simulink model "CLAHEExample"  (R2019b)
settings: Solver=FixedStepDiscrete  StartTime=0.0  StopTime=402*324  FixedStep=1  RelTol=1e-3
PreLoadFcn:
  | % Initialize input image size
  | img = [240 320];
  | 
  | % Number of tiles fixed to 8 x 8
  | numTiles = [8 8];
  | 
  | % Initialize clip limit
  | normClipLimit  = 0.01;
  | 
  | % Number of Bins
  | numBins = 256;
  | 
  | dimI = [240 320] ;
  | 
  | dimTiles = dimI ./ numTiles;
  | 
  | numPixInTile = prod(dimTiles);
  | 
  | minClipLimit = ceil(numPixInTile/numBins);
  | 
  | clipLimit = minClipLimit + round(normClipLimit*(numPixInTile-minClipLimit));
  | 
  | % Initialize value for 1-D lookup table
  | tabVal = uint8(floor(numBins./(1:numBins-1)));
  | 
  | % Initialize wordlength and fractionlength
  | normFact1 = fi(1/(dimTiles(1)*dimTiles(2)/4),0);
  | 
  | normFact2 = fi(1/(prod(dimTiles)/2),0);
  | 
  | normFact3 = fi(1/(prod(dimTiles)),0);
  | 
  | grayxval = (numBins-1)/numPixInTile;
  | fi_grayxval = fi(grayxval,0);
InitFcn:
  | img = imread(get_param('CLAHEExample/inputImage','FileName'));
  | %img = [240 320];
  | numTiles = [8 8];
  | 
  | normClipLimit = str2double(get_param('CLAHEExample/CLAHEHDLAlgorithm','normClipLimit'));
  | 
  | numBins = 256;
  | 
  | dimI = size(img);
  | 
  | dimTiles = dimI ./ numTiles;
  | 
  | numPixInTile = prod(dimTiles);
  | 
  | minClipLimit = ceil(numPixInTile/numBins);
  | 
  | clipLimit = minClipLimit + round(normClipLimit*(numPixInTile-minClipLimit));
  | 
  | tabVal = uint8(floor(numBins./(1:numBins-1)));
  | 
  | normFact1 = fi(1/(dimTiles(1)*dimTiles(2)/4),0);
  | 
  | normFact2 = fi(1/(prod(dimTiles)/2),0);
  | 
  | normFact3 = fi(1/(prod(dimTiles)),0);
  | 
  | grayxval = (numBins-1)/numPixInTile;
  | fi_grayxval = fi(grayxval,0);
libraries: simulink x64, hdlsllib x46, visionhdlutilities x9, visionhdlstatistics x2, visionhdlio x2, visionsources x1
(part 1 of 3)
settings Model: SimulationMode=accelerator  Creator=The MathWorks, Inc.  LastModifiedBy=Bilal
settings OptimizationCC: BlockReduction=off  ConditionallyExecuteInputs=off  DefaultParameterBehavior=Inlined
settings DebuggingCC: AlgebraicLoopMsg=error  SymbolicDimsDataTypeCodeGenerationDiagnostic=none
settings HardwareCC: ProdBitPerPointer=32  ProdBitPerSizeT=32  ProdBitPerPtrDiffT=32  ProdLargestAtomicFloat=None  ProdIntDivRoundTo=Undefined  ProdEndianess=Unspecified  ProdWordSize=32  ProdHWDeviceType=ASIC/FPGA->ASIC/FPGA  TargetBitPerPointer=64  TargetBitPerSizeT=64  TargetBitPerPtrDiffT=64  TargetLongLongMode=on  TargetIntDivRoundTo=Zero  TargetEndianess=LittleEndian  TargetWordSize=64  TargetHWDeviceType=Custom Processor->MATLAB Host Computer  ProdEqTarget=off

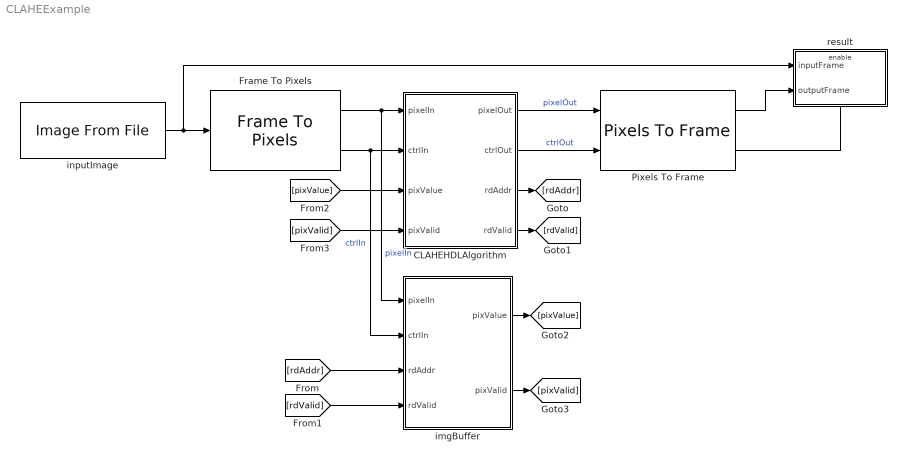
== system CLAHEExample ==
  CLAHEHDLAlgorithm : Subsystem  TreatAsAtomicUnit=on  mask{normClipLimit=0.01}
      mask prompts: normClipLimit "Normalized Clip Limit"
  Frame To Pixels : visionhdlio/Frame To Pixels  NumComponents=1  NumPixels=1  VideoFormat=240p  ActivePixelsPerLine=400  ActiveVideoLines=400  TotalPixelsPerLine=482  TotalVideoLines=430  StartingActiveLine=1  FrontPorch=41  SampleTime=0
      settings: SourceProductName=Vision HDL Toolbox  SourceProductBaseCode=VT
  Pixels To Frame : visionhdlio/Pixels To Frame  NumComponents=1  NumPixels=1  VideoFormat=240p  ActivePixelsPerLine=400  ActiveVideoLines=400  TotalPixelsPerLine=482  TotalVideoLines=430
      settings: SourceProductName=Vision HDL Toolbox  SourceProductBaseCode=VT
  imgBuffer : Subsystem
  inputImage : visionsources/Image From File  Tag=vipblks_nd  FileName=spine240p.tif  Ts=402*324  imagePorts=One multidimensional signal  OutPortLabels=R|G|B  ImageDataType=Inherit from input image  sdImageDataType=uint(8)  Signed=on  WordLength=16  FractionLengthMode=User-defined  FractionLength=15
      settings: SourceProductName=Computer Vision Toolbox
  result : Subsystem
  wires:
  CLAHEHDLAlgorithm/3(rdAddr) -> [rdAddr]
  [pixValue] -> CLAHEHDLAlgorithm/3(pixValue)
  CLAHEHDLAlgorithm/4(rdValid) -> [rdValid]
  inputImage/1 -> result/1(inputFrame), Frame To Pixels/1
  imgBuffer/1(pixValue) -> [pixValue]
  Frame To Pixels/2 -> CLAHEHDLAlgorithm/2(ctrlIn), imgBuffer/2(ctrlIn)  "ctrlIn"
  imgBuffer/2(pixValid) -> [pixValid]
  Pixels To Frame/1 -> result/2(outputFrame)
  CLAHEHDLAlgorithm/2(ctrlOut) -> Pixels To Frame/2  "ctrlOut"
  [pixValid] -> CLAHEHDLAlgorithm/4(pixValid)
  [rdAddr] -> imgBuffer/3(rdAddr)
  Frame To Pixels/1 -> CLAHEHDLAlgorithm/1(pixelIn), imgBuffer/1(pixelIn)  "pixelIn"
  Pixels To Frame/2 -> result/Enable
  [rdValid] -> imgBuffer/4("rdValid ")
  CLAHEHDLAlgorithm/1(pixelOut) -> Pixels To Frame/1  "pixelOut"

== system CLAHEExample/CLAHEHDLAlgorithm ==
  pixelIn : Inport
  ctrlIn : Inport  Port=2
  pixValue : Inport  Port=3
  pixValid : Inport  Port=4
  bilinearInterpolation : Subsystem
  busCreator : Subsystem
  histoEqPipeline : Subsystem
  tileGeneration : Subsystem
  pixelOut : Outport  VectorParamsAs1DForOutWhenUnconnected=off
  ctrlOut : Outport  Port=2  VectorParamsAs1DForOutWhenUnconnected=off
  rdAddr : Outport  Port=3  VectorParamsAs1DForOutWhenUnconnected=off
  rdValid : Outport  Port=4  VectorParamsAs1DForOutWhenUnconnected=off
  wires:
  tileGeneration/2(pixelOut) -> histoEqPipeline/2(pixelIn)
  tileGeneration/3(busPipeline1) -> histoEqPipeline/3(busPipeline1)
  tileGeneration/4(busPipeline2) -> histoEqPipeline/4(busPipeline2)
  tileGeneration/5(resetOut) -> histoEqPipeline/5(reset)
  ctrlIn/1 -> bilinearInterpolation/7(inputCtrl), tileGeneration/2(busIn)
  pixelIn/1 -> tileGeneration/1(pixelIn)
  histoEqPipeline/6(statePipe2) -> bilinearInterpolation/6(statePipe2)
  histoEqPipeline/5(cdfValidPipe2) -> bilinearInterpolation/5(cdfValidPipe2)
  histoEqPipeline/4(cdfValPipe2) -> bilinearInterpolation/4(cdfValPipe2)
  histoEqPipeline/3(statePipe1) -> bilinearInterpolation/3(statePipe1)
  histoEqPipeline/2(cdfValidPipe1) -> bilinearInterpolation/2(cdfValidPipe1)
  histoEqPipeline/1(cdfValPipe1) -> bilinearInterpolation/1(cdfValPipe1)
  bilinearInterpolation/4(pipe2Done) -> [pipe2]
  [pipe2] -> histoEqPipeline/7(state5Pipe2)
  bilinearInterpolation/3(pipe1Done) -> [pipe1]
  [pipe1] -> histoEqPipeline/6(state5Pipe1)
  bilinearInterpolation/5(rdAddr) -> rdAddr/1
  bilinearInterpolation/6(rdValid) -> rdValid/1
  pixValue/1 -> busCreator/1(rd_addr)
  pixValid/1 -> busCreator/2(rd_valid)
  busCreator/1(rdTile1) -> histoEqPipeline/8(state5Bus)
  tileGeneration/1(tileNumber) -> histoEqPipeline/1(tileNumber)
  bilinearInterpolation/1(CLAHEOut) -> pixelOut/1
  bilinearInterpolation/2(ctrlOut) -> ctrlOut/1
  bilinearInterpolation/7(frameDone) -> histoEqPipeline/9(frameDone)

== system CLAHEExample/imgBuffer ==
  pixelIn : Inport
  ctrlIn : Inport  Port=2
  rdAddr : Inport  Port=3
  "rdValid " : Inport  Port=4
  Bus Selector : BusSelector  OutputSignals=vStart,valid
  Delay : Delay  DelayLength=1
  Delay1 : Delay  DelayLength=1
  Delay2 : Delay  DelayLength=1
  HDL Counter : hdlsllib/Sources/HDL Counter  CountType=Count limited  CountInit=0  CountStep=1  CountMax=prod(dimI) - 1  CountFromType=Initial value  CountFrom=0  CountResetPort=on  CountLoadPort=off  CountEnbPort=on  CountDirPort=off  CountDataType=Unsigned  CountWordLen=ceil(log2(prod(dimI)))  CountFracLen=0  CountSampTime=1
      settings: SourceProductName=Simulink
  inputBuffer : hdlsllib/HDL RAMs/Simple Dual Port RAM System  RAMType=Simple dual port  WriteOutputValue=New data  RAMInitialValue=0  SimulateUsing=Code generation
      settings: SourceProductName=Simulink  SourceProductBaseCode=SL
  pixValue : Outport  VectorParamsAs1DForOutWhenUnconnected=off
  pixValid : Outport  Port=2  VectorParamsAs1DForOutWhenUnconnected=off
  wires:
  Delay1/1 -> inputBuffer/1
  Delay/1 -> inputBuffer/3, HDL Counter/2
  Bus Selector/1 -> HDL Counter/1  "<vStart>"
  HDL Counter/1 -> inputBuffer/2
  ctrlIn/1 -> Bus Selector/1
  Bus Selector/2 -> Delay/1  "<valid>"
  pixelIn/1 -> Delay1/1
  "rdValid "/1 -> Delay2/1
  rdAddr/1 -> inputBuffer/4
  inputBuffer/1 -> pixValue/1  "rd_addr"
  Delay2/1 -> pixValid/1  "rd_valid"

== system CLAHEExample/result ==
  inputFrame : Inport
  outputFrame : Inport  Port=2
  Enable : EnablePort
  Input Image : VideoViewer  FigPos=[579 574 378 287]
  Output Image : VideoViewer  FigPos=[579 573 378 285]
  wires:
  outputFrame/1 -> Output Image/1
  inputFrame/1 -> Input Image/1

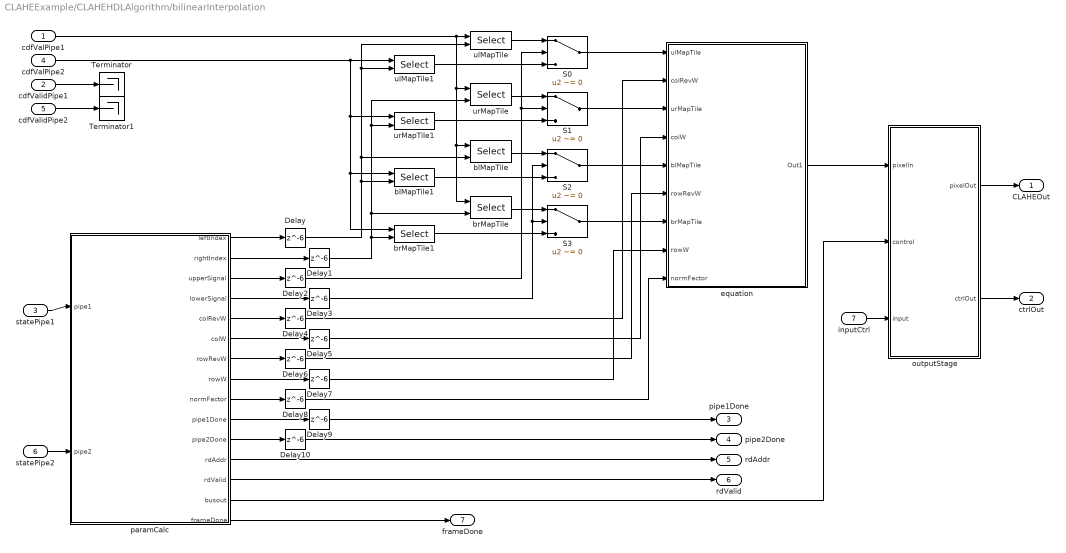
== system CLAHEExample/CLAHEHDLAlgorithm/bilinearInterpolation ==
  cdfValPipe1 : Inport
  cdfValidPipe1 : Inport  Port=2
  statePipe1 : Inport  Port=3
  cdfValPipe2 : Inport  Port=4
  cdfValidPipe2 : Inport  Port=5
  statePipe2 : Inport  Port=6
  inputCtrl : Inport  Port=7
  Delay : Delay  DelayLength=6  InitialCondition=1
  Delay1 : Delay  DelayLength=6  InitialCondition=1
  Delay{2..10} (9 alike) : Delay  DelayLength=6
  S{0..3} (4 alike) : Switch  Criteria=u2 ~= 0
  Terminator : Terminator
  Terminator1 : Terminator
  blMapTile : Selector  InputPortWidth=numTiles(2)  IndexOptions=Index vector (port)  Indices=[1 numTiles(2)]  OutputSizes=1
  blMapTile1 : Selector  InputPortWidth=numTiles(2)  IndexOptions=Index vector (port)  Indices=[1 numTiles(2)]  OutputSizes=1
  brMapTile : Selector  InputPortWidth=numTiles(2)  IndexOptions=Index vector (port)  Indices=[1 numTiles(2)]  OutputSizes=1
  brMapTile1 : Selector  InputPortWidth=numTiles(2)  IndexOptions=Index vector (port)  Indices=[1 numTiles(2)]  OutputSizes=1
  equation : Subsystem
  outputStage : Subsystem
  paramCalc : Subsystem
  ulMapTile : Selector  InputPortWidth=numTiles(2)  IndexOptions=Index vector (port)  Indices=[1 numTiles(2)]  OutputSizes=1
  ulMapTile1 : Selector  InputPortWidth=numTiles(2)  IndexOptions=Index vector (port)  Indices=[1 numTiles(2)]  OutputSizes=1
  urMapTile : Selector  InputPortWidth=numTiles(2)  IndexOptions=Index vector (port)  Indices=[1 numTiles(2)]  OutputSizes=1
  urMapTile1 : Selector  InputPortWidth=numTiles(2)  IndexOptions=Index vector (port)  Indices=[1 numTiles(2)]  OutputSizes=1
  CLAHEOut : Outport  VectorParamsAs1DForOutWhenUnconnected=off
  ctrlOut : Outport  Port=2  VectorParamsAs1DForOutWhenUnconnected=off
  pipe1Done : Outport  Port=3  VectorParamsAs1DForOutWhenUnconnected=off
  pipe2Done : Outport  Port=4  VectorParamsAs1DForOutWhenUnconnected=off
  rdAddr : Outport  Port=5  VectorParamsAs1DForOutWhenUnconnected=off
  rdValid : Outport  Port=6  VectorParamsAs1DForOutWhenUnconnected=off
  frameDone : Outport  Port=7  VectorParamsAs1DForOutWhenUnconnected=off
  wires:
  S0/1 -> equation/1(ulMapTile)
  S1/1 -> equation/3(urMapTile)
  S2/1 -> equation/5(blMapTile)
  S3/1 -> equation/7(brMapTile)
  urMapTile/1 -> S1/1
  ulMapTile/1 -> S0/1
  blMapTile/1 -> S2/1
  brMapTile/1 -> S3/1
  ulMapTile1/1 -> S0/3
  urMapTile1/1 -> S1/3
  blMapTile1/1 -> S2/3
  brMapTile1/1 -> S3/3
  cdfValPipe1/1 -> brMapTile/1, blMapTile/1, urMapTile/1, ulMapTile/1
  paramCalc/1(leftIndex) -> Delay/1
  paramCalc/2(rightIndex) -> Delay1/1
  paramCalc/3(upperSignal) -> Delay2/1
  paramCalc/4(lowerSignal) -> Delay3/1
  paramCalc/6(colW) -> Delay5/1
  paramCalc/5(colRevW) -> Delay4/1
  paramCalc/8(rowW) -> Delay7/1
  paramCalc/7(rowRevW) -> Delay6/1
  paramCalc/9(normFactor) -> Delay8/1
  statePipe1/1 -> paramCalc/1(pipe1)
  statePipe2/1 -> paramCalc/2(pipe2)
  paramCalc/10(pipe1Done) -> Delay9/1
  paramCalc/11(pipe2Done) -> Delay10/1
  paramCalc/12(rdAddr) -> rdAddr/1
  paramCalc/13(rdValid) -> rdValid/1
  cdfValidPipe2/1 -> Terminator1/1
  Delay/1 -> blMapTile1/2, blMapTile/2, ulMapTile1/2, ulMapTile/2
  Delay1/1 -> brMapTile/2, urMapTile/2, urMapTile1/2, brMapTile1/2
  Delay3/1 -> S3/2, S2/2
  Delay2/1 -> S1/2, S0/2
  Delay4/1 -> equation/2(colRevW)
  Delay5/1 -> equation/4(colW)
  Delay7/1 -> equation/8(rowW)
  Delay6/1 -> equation/6(rowRevW)
  Delay8/1 -> equation/9(normFactor)
  Delay10/1 -> pipe2Done/1
  Delay9/1 -> pipe1Done/1
  cdfValidPipe1/1 -> Terminator/1
  cdfValPipe2/1 -> brMapTile1/1, blMapTile1/1, urMapTile1/1, ulMapTile1/1
  inputCtrl/1 -> outputStage/3("input ")
  paramCalc/14(busout) -> outputStage/2("control ")
  paramCalc/15(frameDone) -> frameDone/1
  equation/1(Out1) -> outputStage/1(pixelIn)
  outputStage/1(pixelOut) -> CLAHEOut/1
  outputStage/2(ctrlOut) -> ctrlOut/1

== system CLAHEExample/CLAHEHDLAlgorithm/busCreator ==
  rd_addr : Inport
  rd_valid : Inport  Port=2
  Bus Creator : BusCreator  Inputs=5
  Constant : Constant  OutDataTypeStr=fixdt(0,ceil(log2(numPixInTile)),0)  SampleTime=-1
  Constant1 : Constant  Value=0  OutDataTypeStr=uint8  SampleTime=-1
  Constant2 : Constant  Value=0  OutDataTypeStr=boolean  SampleTime=-1
  rdTile1 : Outport  VectorParamsAs1DForOutWhenUnconnected=off
  wires:
  rd_addr/1 -> Bus Creator/4  "rd_addr"
  Constant1/1 -> Bus Creator/2  "wr_addr"
  Bus Creator/1 -> rdTile1/1
  Constant2/1 -> Bus Creator/3  "wr_en"
  Constant/1 -> Bus Creator/1  "histVal"
  rd_valid/1 -> Bus Creator/5  "rd_valid"

== system CLAHEExample/CLAHEHDLAlgorithm/histoEqPipeline ==
  tileNumber : Inport
  pixelIn : Inport  Port=2
  busPipeline1 : Inport  Port=3
  busPipeline2 : Inport  Port=4
  reset : Inport  Port=5
  state5Pipe1 : Inport  Port=6
  state5Pipe2 : Inport  Port=7
  state5Bus : Inport  Port=8
  frameDone : Inport  Port=9
  Constant : Constant  Value=1:numTiles(2)  OutDataTypeStr=uint8  SampleTime=-1
  histPipe1 : Subsystem  TreatAsAtomicUnit=on
  histPipe2 : Subsystem  TreatAsAtomicUnit=on
  cdfValPipe1 : Outport  VectorParamsAs1DForOutWhenUnconnected=off
  cdfValidPipe1 : Outport  Port=2  VectorParamsAs1DForOutWhenUnconnected=off
  statePipe1 : Outport  Port=3  VectorParamsAs1DForOutWhenUnconnected=off
  cdfValPipe2 : Outport  Port=4  VectorParamsAs1DForOutWhenUnconnected=off
  cdfValidPipe2 : Outport  Port=5  VectorParamsAs1DForOutWhenUnconnected=off
  statePipe2 : Outport  Port=6  VectorParamsAs1DForOutWhenUnconnected=off
  wires:
  pixelIn/1 -> histPipe2/3(pixelIn), histPipe1/3(pixelIn)
  reset/1 -> histPipe2/5(reset), histPipe1/5(reset)
  busPipeline1/1 -> histPipe1/4(busIn1)
  busPipeline2/1 -> histPipe2/4(busIn1)
  histPipe1/1(cdfVal) -> cdfValPipe1/1
  histPipe1/2(cdfValid) -> cdfValidPipe1/1
  histPipe1/3(pipeState) -> statePipe1/1
  histPipe2/3(pipeState) -> statePipe2/1
  state5Bus/1 -> histPipe1/7(state5Bus), histPipe2/7(state5Bus)
  state5Pipe1/1 -> histPipe1/6(state5Done)
  state5Pipe2/1 -> histPipe2/6(state5Done)
  tileNumber/1 -> histPipe2/2(tileNumber), histPipe1/2(tileNumber)
  Constant/1 -> histPipe2/1(index), histPipe1/1(index)
  frameDone/1 -> histPipe2/8(frameDone), histPipe1/8(frameDone)
  histPipe2/2(cdfValid) -> cdfValidPipe2/1
  histPipe2/1(cdfVal) -> cdfValPipe2/1

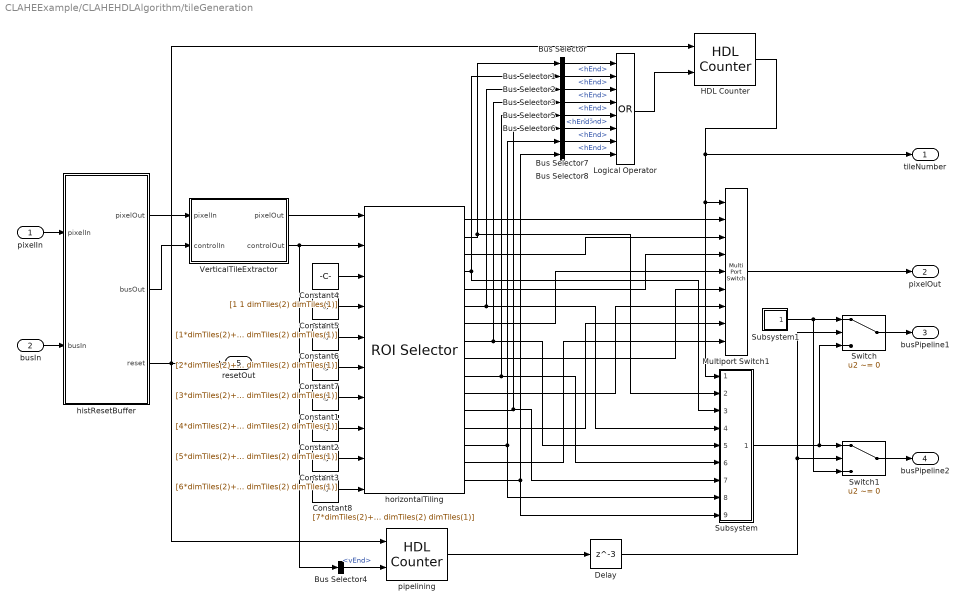
== system CLAHEExample/CLAHEHDLAlgorithm/tileGeneration ==
  pixelIn : Inport
  busIn : Inport  Port=2
  Bus Selector{,1..3,5..8} (8 alike) : BusSelector  OutputSignals=hEnd
  Bus Selector4 : BusSelector  OutputSignals=vEnd
  Constant1 : Constant  Value=[4*dimTiles(2)+1 1 dimTiles(2) dimTiles(1)]  OutDataTypeStr=fixdt(0,ceil(log2(dimI(2))),0)  SampleTime=-1
  Constant2 : Constant  Value=[5*dimTiles(2)+1 1 dimTiles(2) dimTiles(1)]  OutDataTypeStr=fixdt(0,ceil(log2(dimI(2))),0)  SampleTime=-1
  Constant3 : Constant  Value=[6*dimTiles(2)+1 1 dimTiles(2) dimTiles(1)]  OutDataTypeStr=fixdt(0,ceil(log2(dimI(2))),0)  SampleTime=-1
  Constant4 : Constant  Value=[1 1 dimTiles(2) dimTiles(1)]  OutDataTypeStr=fixdt(0,ceil(log2(dimI(2))),0)  SampleTime=-1
  Constant5 : Constant  Value=[1*dimTiles(2)+1 1 dimTiles(2) dimTiles(1)]  OutDataTypeStr=fixdt(0,ceil(log2(dimI(2))),0)  SampleTime=-1
  Constant6 : Constant  Value=[2*dimTiles(2)+1 1 dimTiles(2) dimTiles(1)]  OutDataTypeStr=fixdt(0,ceil(log2(dimI(2))),0)  SampleTime=-1
  Constant7 : Constant  Value=[3*dimTiles(2)+1 1 dimTiles(2) dimTiles(1)]  OutDataTypeStr=fixdt(0,ceil(log2(dimI(2))),0)  SampleTime=-1
  Constant8 : Constant  Value=[7*dimTiles(2)+1 1 dimTiles(2) dimTiles(1)]  OutDataTypeStr=fixdt(0,ceil(log2(dimI(2))),0)  SampleTime=-1
  Delay : Delay  DelayLength=3
  HDL Counter : hdlsllib/Sources/HDL Counter  CountType=Count limited  CountInit=1  CountStep=1  CountMax=numTiles(2)  CountFromType=Initial value  CountFrom=1  CountResetPort=on  CountLoadPort=off  CountEnbPort=on  CountDirPort=off  CountDataType=Unsigned  CountWordLen=4  CountFracLen=0  CountSampTime=1
      settings: SourceProductName=Simulink
  Logical Operator : Logic  Operator=OR  Inputs=8  AllPortsSameDT=off  OutDataTypeStr=boolean
  Multiport Switch1 : MultiPortSwitch  Inputs=8
  Subsystem : Subsystem
  Subsystem1 : Subsystem
  Switch : Switch  Criteria=u2 ~= 0
  Switch1 : Switch  Criteria=u2 ~= 0
  VerticalTileExtractor : Subsystem
  histResetBuffer : Subsystem
  horizontalTiling : visionhdlutilities/ROI Selector  RegionsSource=Input port  NumberOfRegions=8  Regions=[100 100 50 50]  SimulateUsing=Code generation
      settings: SourceProductName=Vision HDL Toolbox  SourceProductBaseCode=VT
  pipelining : hdlsllib/Sources/HDL Counter  CountType=Count limited  CountInit=0  CountStep=1  CountMax=1  CountFromType=Initial value  CountFrom=0  CountResetPort=on  CountLoadPort=off  CountEnbPort=on  CountDirPort=off  CountDataType=Unsigned  CountWordLen=4  CountFracLen=0  CountSampTime=1
      settings: SourceProductName=Simulink
  tileNumber : Outport  VectorParamsAs1DForOutWhenUnconnected=off
  pixelOut : Outport  Port=2  VectorParamsAs1DForOutWhenUnconnected=off
  busPipeline1 : Outport  Port=3  VectorParamsAs1DForOutWhenUnconnected=off
  busPipeline2 : Outport  Port=4  VectorParamsAs1DForOutWhenUnconnected=off
  resetOut : Outport  Port=5  VectorParamsAs1DForOutWhenUnconnected=off
  wires:
  pixelIn/1 -> histResetBuffer/1(pixelIn)
  busIn/1 -> histResetBuffer/2(busIn)
  VerticalTileExtractor/2(controlOut) -> Bus Selector4/1, horizontalTiling/2
  Constant6/1 -> horizontalTiling/5
  Constant4/1 -> horizontalTiling/3
  Constant7/1 -> horizontalTiling/6
  Constant5/1 -> horizontalTiling/4
  histResetBuffer/1(pixelOut) -> VerticalTileExtractor/1(pixelIn)
  histResetBuffer/2(busOut) -> VerticalTileExtractor/2(controlIn)
  HDL Counter/1 -> tileNumber/1, Subsystem/1(In1), Multiport Switch1/1
  Logical Operator/1 -> HDL Counter/2
  Bus Selector/1 -> Logical Operator/1  "<hEnd>"
  Bus Selector1/1 -> Logical Operator/2  "<hEnd>"
  Bus Selector2/1 -> Logical Operator/3  "<hEnd>"
  Bus Selector3/1 -> Logical Operator/4  "<hEnd>"
  histResetBuffer/3(reset) -> pipelining/1, resetOut/1, HDL Counter/1
  Multiport Switch1/1 -> pixelOut/1
  Bus Selector4/1 -> pipelining/2  "<vEnd>"
  Subsystem/1(Out1) -> Switch/3, Switch1/1
  Switch/1 -> busPipeline1/1
  pipelining/1 -> Delay/1
  Subsystem1/1(Out1) -> Switch1/3, Switch/1
  Switch1/1 -> busPipeline2/1
  Delay/1 -> Switch/2, Switch1/2
  Constant3/1 -> horizontalTiling/9
  Constant8/1 -> horizontalTiling/10
  Constant1/1 -> horizontalTiling/7
  Constant2/1 -> horizontalTiling/8
  horizontalTiling/1 -> Multiport Switch1/2
  horizontalTiling/3 -> Multiport Switch1/3
  horizontalTiling/5 -> Multiport Switch1/4
  horizontalTiling/7 -> Multiport Switch1/5
  horizontalTiling/9 -> Multiport Switch1/6
  horizontalTiling/11 -> Multiport Switch1/7
  horizontalTiling/13 -> Multiport Switch1/8
  horizontalTiling/15 -> Multiport Switch1/9
  Bus Selector7/1 -> Logical Operator/7  "<hEnd>"
  Bus Selector8/1 -> Logical Operator/8  "<hEnd>"
  Bus Selector5/1 -> Logical Operator/5  "<hEnd>"
  Bus Selector6/1 -> Logical Operator/6  "<hEnd>"
  horizontalTiling/2 -> Subsystem/2(In2), Bus Selector/1
  horizontalTiling/4 -> Subsystem/3(In3), Bus Selector1/1
  horizontalTiling/6 -> Subsystem/4(In4), Bus Selector2/1
  horizontalTiling/8 -> Subsystem/5(In5), Bus Selector3/1
  horizontalTiling/10 -> Subsystem/6(In6), Bus Selector5/1
  horizontalTiling/12 -> Subsystem/7(In7), Bus Selector6/1
  horizontalTiling/14 -> Bus Selector7/1, Subsystem/8(In8)
  horizontalTiling/16 -> Subsystem/9(In9), Bus Selector8/1
  VerticalTileExtractor/1(pixelOut) -> horizontalTiling/1

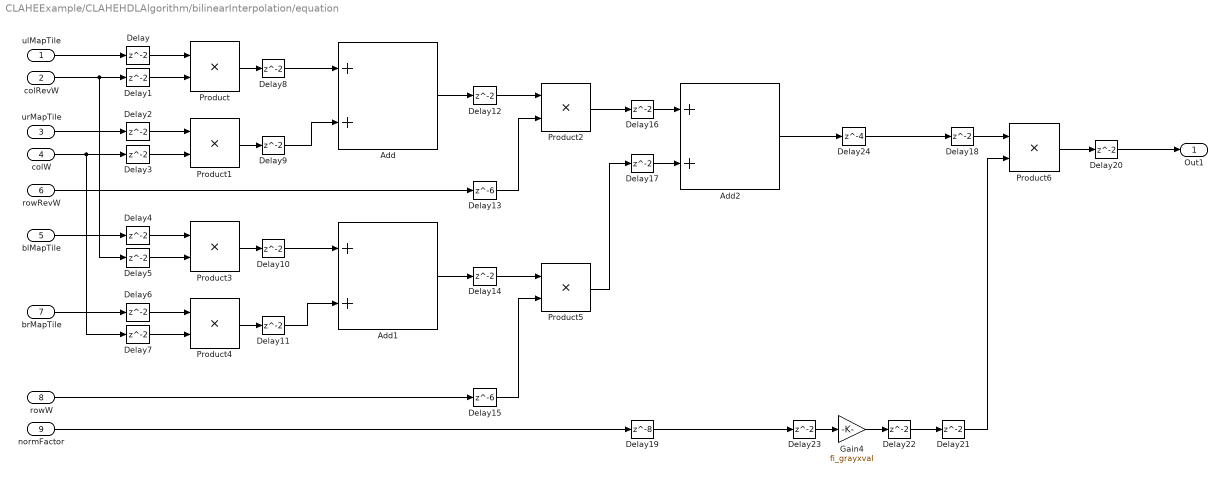
== system CLAHEExample/CLAHEHDLAlgorithm/bilinearInterpolation/equation ==
  ulMapTile : Inport
  colRevW : Inport  Port=2
  urMapTile : Inport  Port=3
  colW : Inport  Port=4
  blMapTile : Inport  Port=5
  rowRevW : Inport  Port=6
  brMapTile : Inport  Port=7
  rowW : Inport  Port=8
  normFactor : Inport  Port=9
  Add : Sum
  Add1 : Sum
  Add2 : Sum
  Delay{,1..12,14,16..18,20..23} (21 alike) : Delay
  Delay13 : Delay  DelayLength=6
  Delay15 : Delay  DelayLength=6
  Delay19 : Delay  DelayLength=8
  Delay24 : Delay  DelayLength=4
  Gain4 : Gain  Gain=fi_grayxval  RndMeth=Round  OutDataTypeStr=Inherit: Same as input  LockScale=on
  Product{,1..5} (6 alike) : Product
  Product6 : Product  OutDataTypeStr=uint8  RndMeth=Round  SaturateOnIntegerOverflow=on  LockScale=on
  Out1 : Outport  VectorParamsAs1DForOutWhenUnconnected=off
  wires:
  Product1/1 -> Delay9/1
  Product/1 -> Delay8/1
  Add/1 -> Delay12/1
  Product3/1 -> Delay10/1
  rowW/1 -> Delay15/1
  Product4/1 -> Delay11/1
  Add1/1 -> Delay14/1
  Product2/1 -> Delay16/1
  Product5/1 -> Delay17/1
  normFactor/1 -> Delay19/1
  Delay24/1 -> Delay18/1
  Product6/1 -> Delay20/1
  ulMapTile/1 -> Delay/1
  urMapTile/1 -> Delay2/1
  blMapTile/1 -> Delay4/1
  brMapTile/1 -> Delay6/1
  Delay/1 -> Product/1
  Delay1/1 -> Product/2
  Delay2/1 -> Product1/1
  Delay3/1 -> Product1/2
  Delay4/1 -> Product3/1
  Delay5/1 -> Product3/2
  Delay7/1 -> Product4/2
  Delay6/1 -> Product4/1
  Delay8/1 -> Add/1
  Delay9/1 -> Add/2
  Delay10/1 -> Add1/1
  Delay11/1 -> Add1/2
  Delay12/1 -> Product2/1
  Delay13/1 -> Product2/2
  Delay14/1 -> Product5/1
  Delay15/1 -> Product5/2
  Delay16/1 -> Add2/1
  Delay17/1 -> Add2/2
  Delay18/1 -> Product6/1
  colRevW/1 -> Delay5/1, Delay1/1
  colW/1 -> Delay7/1, Delay3/1
  rowRevW/1 -> Delay13/1
  Delay19/1 -> Delay23/1
  Delay21/1 -> Product6/2
  Add2/1 -> Delay24/1
  Delay22/1 -> Delay21/1
  Delay20/1 -> Out1/1
  Delay23/1 -> Gain4/1
  Gain4/1 -> Delay22/1

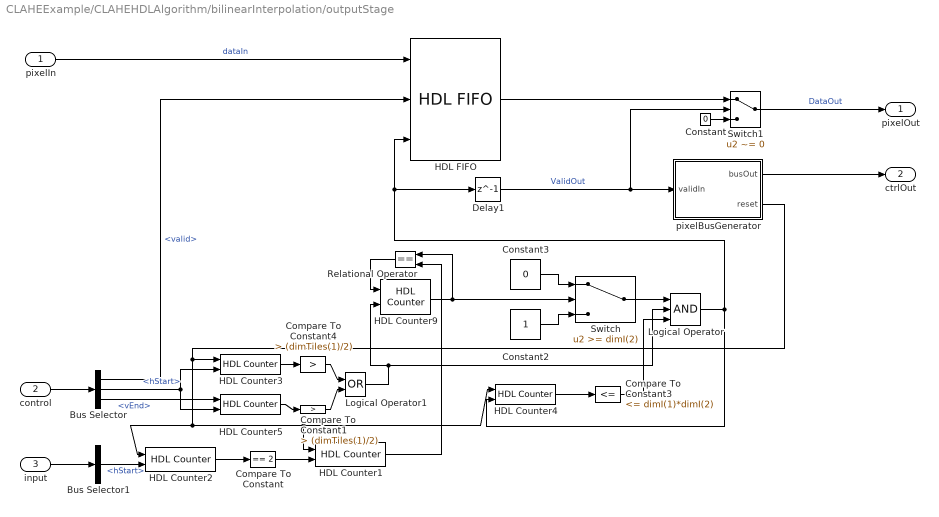
== system CLAHEExample/CLAHEHDLAlgorithm/bilinearInterpolation/outputStage ==
  pixelIn : Inport
  "control " : Inport  Port=2
  "input " : Inport  Port=3
  Bus Selector : BusSelector  OutputSignals=valid,hStart,vEnd
  Bus Selector1 : BusSelector  OutputSignals=hStart
  Compare To Constant : simulink/Logic and Bit Operations/Compare To Constant  relop===  const=2  OutDataTypeStr=boolean
  Compare To Constant1 : simulink/Logic and Bit Operations/Compare To Constant  relop=>  const=(dimTiles(1)/2)  OutDataTypeStr=boolean
  Compare To Constant3 : simulink/Logic and Bit Operations/Compare To Constant  relop=<=  const=dimI(1)*dimI(2)  OutDataTypeStr=boolean
  Compare To Constant4 : simulink/Logic and Bit Operations/Compare To Constant  relop=>  const=(dimTiles(1)/2)  OutDataTypeStr=boolean
  Constant : Constant  Value=0  OutDataTypeStr=Inherit: Inherit via back propagation  SampleTime=-1
  Constant2 : Constant  OutDataTypeStr=boolean  SampleTime=-1
  Constant3 : Constant  Value=0  OutDataTypeStr=boolean  SampleTime=-1
  Delay1 : Delay  DelayLength=1
  HDL Counter1 : hdlsllib/Sources/HDL Counter  CountType=Free running  CountInit=-1  CountStep=1  CountMax=29  CountFromType=Initial value  CountFrom=-1  CountResetPort=on  CountLoadPort=off  CountEnbPort=on  CountDirPort=off  CountDataType=Signed  CountWordLen=ceil(log2(dimI(2)*2))  CountFracLen=0  CountSampTime=1
      settings: SourceProductName=Simulink
  HDL Counter2 : hdlsllib/Sources/HDL Counter  CountType=Free running  CountInit=0  CountStep=1  CountMax=29  CountFromType=Initial value  CountFrom=0  CountResetPort=on  CountLoadPort=off  CountEnbPort=on  CountDirPort=off  CountDataType=Unsigned  CountWordLen=ceil(log2(dimI(2)*dimI(1)*3))  CountFracLen=0  CountSampTime=1
      settings: SourceProductName=Simulink
  HDL Counter3 : hdlsllib/Sources/HDL Counter  CountType=Free running  CountInit=0  CountStep=1  CountMax=25  CountFromType=Initial value  CountFrom=0  CountResetPort=on  CountLoadPort=off  CountEnbPort=on  CountDirPort=off  CountDataType=Unsigned  CountWordLen=ceil(log2(dimI(1)+2))  CountFracLen=0  CountSampTime=1
      settings: SourceProductName=Simulink
  HDL Counter4 : hdlsllib/Sources/HDL Counter  CountType=Free running  CountInit=0  CountStep=1  CountMax=25  CountFromType=Initial value  CountFrom=0  CountResetPort=on  CountLoadPort=off  CountEnbPort=on  CountDirPort=off  CountDataType=Unsigned  CountWordLen=ceil(log2(dimI(2)*dimI(1)*1.5))  CountFracLen=0  CountSampTime=1
      settings: SourceProductName=Simulink
  HDL Counter5 : hdlsllib/Sources/HDL Counter  CountType=Free running  CountInit=0  CountStep=1  CountMax=25  CountFromType=Initial value  CountFrom=0  CountResetPort=on  CountLoadPort=off  CountEnbPort=on  CountDirPort=off  CountDataType=Unsigned  CountWordLen=ceil(log2(dimI(1)+2))  CountFracLen=0  CountSampTime=1
      settings: SourceProductName=Simulink
  HDL Counter9 : hdlsllib/Sources/HDL Counter  CountType=Free running  CountInit=0  CountStep=1  CountMax=29  CountFromType=Initial value  CountFrom=0  CountResetPort=on  CountLoadPort=off  CountEnbPort=on  CountDirPort=off  CountDataType=Unsigned  CountWordLen=ceil(log2(dimI(2)*2))  CountFracLen=0  CountSampTime=1
      settings: SourceProductName=Simulink
  HDL FIFO : hdlsllib/HDL RAMs/HDL FIFO  fifo_size=(dimTiles(1)*1.5)*dimI(2)  mode=Classic  ratio=1  push_msg=Warning  pop_msg=Warning  show_empty=off  show_full=off  show_num=off  LabelModeActiveChoice_Mode=Classic
      settings: SourceProductName=Simulink  SourceProductBaseCode=SL
  Logical Operator : Logic  Inputs=3  AllPortsSameDT=off  OutDataTypeStr=boolean
  Logical Operator1 : Logic  Operator=OR  AllPortsSameDT=off  OutDataTypeStr=boolean
  Relational Operator : RelationalOperator  Operator===  OutDataTypeStr=boolean  RndMeth=Nearest
  Switch : Switch  Threshold=dimI(2)
  Switch1 : Switch  Criteria=u2 ~= 0
  pixelBusGenerator : Subsystem  mask{hEnd=dimI(2)-1, vEnd=dimI(1)*dimI(2) - 1}
      mask prompts: hEnd "hEnd Count"; vEnd "vEnd Count"
      mask DialogControl DescGroupVar Prompt: Counter Values
  pixelOut : Outport  VectorParamsAs1DForOutWhenUnconnected=off
  ctrlOut : Outport  Port=2  VectorParamsAs1DForOutWhenUnconnected=off
  wires:
  pixelIn/1 -> HDL FIFO/1  "dataIn"
  "control "/1 -> Bus Selector/1
  Bus Selector/1 -> HDL FIFO/2  "<valid>"
  Switch1/1 -> pixelOut/1  "DataOut"
  Constant3/1 -> Switch/1
  Switch/1 -> Logical Operator/1
  Constant2/1 -> Switch/3
  HDL Counter9/1 -> Relational Operator/1, Switch/2
  pixelBusGenerator/2(reset) -> HDL Counter3/1, HDL Counter2/1, HDL Counter1/1, HDL Counter4/1
  HDL FIFO/1 -> Switch1/1
  Constant/1 -> Switch1/3
  Logical Operator/1 -> HDL Counter4/2, HDL FIFO/3, Delay1/1
  pixelBusGenerator/1(busOut) -> ctrlOut/1
  Delay1/1 -> Switch1/2, pixelBusGenerator/1(validIn)  "ValidOut"
  "input "/1 -> Bus Selector1/1
  HDL Counter1/1 -> Relational Operator/2
  Bus Selector1/1 -> HDL Counter2/2  "<hStart>"
  HDL Counter2/1 -> Compare To Constant/1
  Compare To Constant/1 -> HDL Counter1/2
  Relational Operator/1 -> HDL Counter9/1
  Bus Selector/2 -> HDL Counter3/2, HDL Counter5/2  "<hStart>"
  Bus Selector/3 -> HDL Counter5/1  "<vEnd>"
  Logical Operator1/1 -> Logical Operator/2, HDL Counter9/2
  HDL Counter3/1 -> Compare To Constant4/1
  Compare To Constant4/1 -> Logical Operator1/1
  HDL Counter5/1 -> Compare To Constant1/1
  Compare To Constant1/1 -> Logical Operator1/2
  HDL Counter4/1 -> Compare To Constant3/1
  Compare To Constant3/1 -> Logical Operator/3

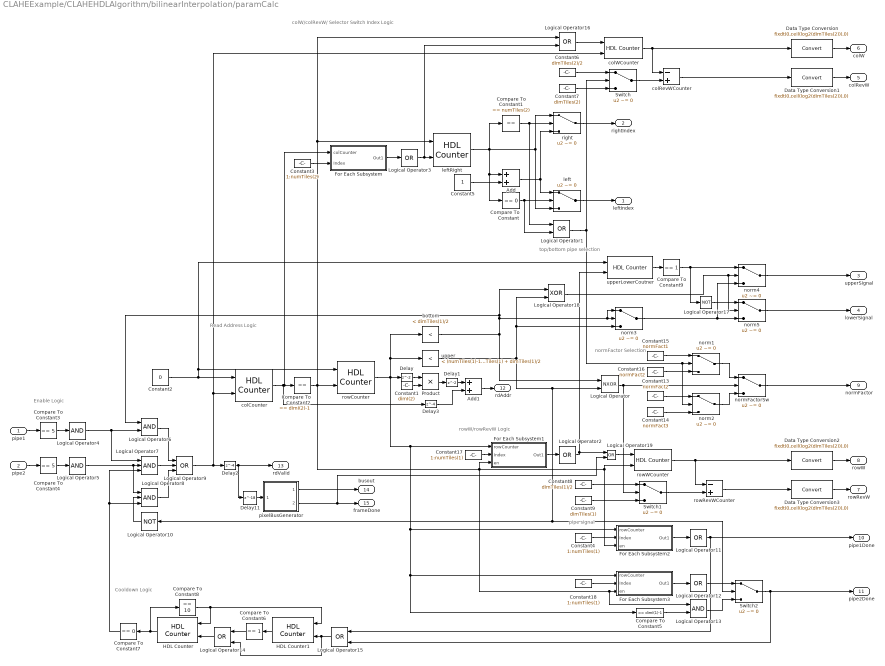
== system CLAHEExample/CLAHEHDLAlgorithm/bilinearInterpolation/paramCalc ==
  note: Enable Logic
  note: Cooldown Logic
  note: pipe signal
  note: rowW/rowRevW Logic
  note: colW/colRevW/ Selector Switch Index Logic
  note: top/bottom pipe selection
  note: normFactor Selection
  note: Read Address Logic
  pipe1 : Inport
  pipe2 : Inport  Port=2
  Add : Sum  OutDataTypeStr=uint8
  Add1 : Sum  OutDataTypeStr=fixdt(0,ceil(log2(prod(dimI))),0)
  Compare To Constant : simulink/Logic and Bit Operations/Compare To Constant  relop===  const=0  OutDataTypeStr=boolean
  Compare To Constant1 : simulink/Logic and Bit Operations/Compare To Constant  relop===  const=numTiles(2)  OutDataTypeStr=boolean
  Compare To Constant2 : simulink/Logic and Bit Operations/Compare To Constant  relop===  const=dimI(2)-1  OutDataTypeStr=boolean
  Compare To Constant3 : simulink/Logic and Bit Operations/Compare To Constant  relop===  const=5  OutDataTypeStr=boolean
  Compare To Constant4 : simulink/Logic and Bit Operations/Compare To Constant  relop===  const=5  OutDataTypeStr=boolean
  Compare To Constant5 : simulink/Logic and Bit Operations/Compare To Constant  relop===  const=dimI(1)-1  OutDataTypeStr=boolean
  Compare To Constant6 : simulink/Logic and Bit Operations/Compare To Constant  relop===  const=1  OutDataTypeStr=boolean
  Compare To Constant7 : simulink/Logic and Bit Operations/Compare To Constant  relop===  const=0  OutDataTypeStr=boolean
  Compare To Constant8 : simulink/Logic and Bit Operations/Compare To Constant  relop===  const=10  OutDataTypeStr=boolean
  Compare To Constant9 : simulink/Logic and Bit Operations/Compare To Constant  relop===  const=1  OutDataTypeStr=boolean
  Constant1 : Constant  Value=dimI(2)  OutDataTypeStr=fixdt(0,ceil(log2(dimI(2))),0)  SampleTime=-1
  Constant13 : Constant  Value=normFact2  SampleTime=-1  LockScale=on
  Constant14 : Constant  Value=normFact3  SampleTime=-1  LockScale=on
  Constant15 : Constant  Value=normFact1  SampleTime=-1  LockScale=on
  Constant16 : Constant  Value=normFact2  SampleTime=-1  LockScale=on
  Constant17 : Constant  Value=1:numTiles(1)  OutDataTypeStr=uint8  SampleTime=-1
  Constant18 : Constant  Value=1:numTiles(1)  OutDataTypeStr=uint8  SampleTime=-1
  Constant2 : Constant  Value=0  OutDataTypeStr=boolean  SampleTime=-1
  Constant3 : Constant  Value=1:numTiles(2)  OutDataTypeStr=uint8  SampleTime=-1
  Constant4 : Constant  Value=1:numTiles(1)  OutDataTypeStr=uint8  SampleTime=-1
  Constant5 : Constant  OutDataTypeStr=boolean  SampleTime=-1
  Constant6 : Constant  Value=dimTiles(2)/2  OutDataTypeStr=uint8  SampleTime=-1
  Constant7 : Constant  Value=dimTiles(2)  OutDataTypeStr=uint8  SampleTime=-1
  Constant8 : Constant  Value=dimTiles(1)/2  OutDataTypeStr=uint8  SampleTime=-1
  Constant9 : Constant  Value=dimTiles(1)  OutDataTypeStr=uint8  SampleTime=-1
  Data Type Conversion{,1..3} (4 alike) : DataTypeConversion  OutDataTypeStr=fixdt(0,ceil(log2(dimTiles(2))),0)
  Delay : Delay
  Delay1 : Delay
  Delay11 : Delay  DelayLength=18
  Delay2 : Delay  DelayLength=4
  Delay3 : Delay  DelayLength=4
  For Each Subsystem : Subsystem  TreatAsAtomicUnit=on
  For Each Subsystem1 : Subsystem  TreatAsAtomicUnit=on
  For Each Subsystem2 : Subsystem  TreatAsAtomicUnit=on
  For Each Subsystem3 : Subsystem  TreatAsAtomicUnit=on
  HDL Counter : hdlsllib/Sources/HDL Counter  CountType=Free running  CountInit=0  CountStep=1  CountMax=5  CountFromType=Initial value  CountFrom=0  CountResetPort=on  CountLoadPort=off  CountEnbPort=on  CountDirPort=off  CountDataType=Unsigned  CountWordLen=8  CountFracLen=0  CountSampTime=1
      settings: SourceProductName=Simulink
  HDL Counter1 : hdlsllib/Sources/HDL Counter  CountType=Count limited  CountInit=0  CountStep=1  CountMax=1  CountFromType=Initial value  CountFrom=0  CountResetPort=on  CountLoadPort=off  CountEnbPort=on  CountDirPort=off  CountDataType=Unsigned  CountWordLen=1  CountFracLen=0  CountSampTime=1
      settings: SourceProductName=Simulink
  Logical Operator : Logic  Operator=NXOR  AllPortsSameDT=off  OutDataTypeStr=boolean
  Logical Operator{1,14..16,19} (5 alike) : Logic  Operator=OR  AllPortsSameDT=off  OutDataTypeStr=boolean
  Logical Operator10 : Logic  Operator=NOT  AllPortsSameDT=off  OutDataTypeStr=boolean
  Logical Operator{2..3,11..12} (4 alike) : Logic  Operator=OR  Inputs=1  AllPortsSameDT=off  OutDataTypeStr=boolean
  Logical Operator13 : Logic  AllPortsSameDT=off  OutDataTypeStr=boolean
  Logical Operator17 : Logic  Operator=NOT  Inputs=1  AllPortsSameDT=off  OutDataTypeStr=boolean
  Logical Operator18 : Logic  Operator=XOR  AllPortsSameDT=off  OutDataTypeStr=boolean
  Logical Operator4 : Logic  Inputs=1  AllPortsSameDT=off  OutDataTypeStr=boolean
  Logical Operator5 : Logic  Inputs=1  AllPortsSameDT=off  OutDataTypeStr=boolean
  Logical Operator6 : Logic  AllPortsSameDT=off  OutDataTypeStr=boolean
  Logical Operator7 : Logic  Inputs=3  AllPortsSameDT=off  OutDataTypeStr=boolean
  Logical Operator8 : Logic  Inputs=3  AllPortsSameDT=off  OutDataTypeStr=boolean
  Logical Operator9 : Logic  Operator=OR  Inputs=3  AllPortsSameDT=off  OutDataTypeStr=boolean
  Product : Product
  Switch : Switch  Criteria=u2 ~= 0
  Switch1 : Switch  Criteria=u2 ~= 0
  Switch2 : Switch  Criteria=u2 ~= 0
  bottom : simulink/Logic and Bit Operations/Compare To Constant  relop=<  const=dimTiles(1)/2  OutDataTypeStr=boolean
  colCounter : hdlsllib/Sources/HDL Counter  CountType=Count limited  CountInit=0  CountStep=1  CountMax=dimI(2)-1  CountFromType=Initial value  CountFrom=0  CountResetPort=on  CountLoadPort=off  CountEnbPort=on  CountDirPort=off  CountDataType=Unsigned  CountWordLen=ceil(log2(dimI(2)))  CountFracLen=0  CountSampTime=1
      settings: SourceProductName=Simulink
  colRevWCounter : Sum  Inputs=-+
  colWCounter : hdlsllib/Sources/HDL Counter  CountType=Free running  CountInit=0  CountStep=1  CountMax=25  CountFromType=Initial value  CountFrom=0  CountResetPort=on  CountLoadPort=off  CountEnbPort=on  CountDirPort=off  CountDataType=Unsigned  CountWordLen=8  CountFracLen=0  CountSampTime=1
      settings: SourceProductName=Simulink
  left : Switch  Criteria=u2 ~= 0
  leftRight : hdlsllib/Sources/HDL Counter  CountType=Count limited  CountInit=0  CountStep=1  CountMax=numTiles(2)  CountFromType=Initial value  CountFrom=0  CountResetPort=on  CountLoadPort=off  CountEnbPort=on  CountDirPort=off  CountDataType=Unsigned  CountWordLen=ceil(log2(numTiles(2)))+1  CountFracLen=0  CountSampTime=1
      settings: SourceProductName=Simulink
  norm{1..5} (5 alike) : Switch  Criteria=u2 ~= 0
  normFactorSw : Switch  Criteria=u2 ~= 0
  pixelBusGenerator : Subsystem  mask{hEnd=dimI(2)-1, vEnd=dimI(1)*dimI(2) - 1}
      mask prompts: hEnd "hEnd Count"; vEnd "vEnd Count"
      mask DialogControl DescGroupVar Prompt: Counter Values
  right : Switch  Criteria=u2 ~= 0
  rowCounter : hdlsllib/Sources/HDL Counter  CountType=Count limited  CountInit=0  CountStep=1  CountMax=dimI(1)-1  CountFromType=Initial value  CountFrom=0  CountResetPort=on  CountLoadPort=off  CountEnbPort=on  CountDirPort=off  CountDataType=Unsigned  CountWordLen=ceil(log2(dimI(1)))  CountFracLen=0  CountSampTime=1
      settings: SourceProductName=Simulink
  rowRevWCounter : Sum  Inputs=-+
  rowWCounter : hdlsllib/Sources/HDL Counter  CountType=Free running  CountInit=0  CountStep=1  CountMax=25  CountFromType=Initial value  CountFrom=0  CountResetPort=on  CountLoadPort=off  CountEnbPort=on  CountDirPort=off  CountDataType=Unsigned  CountWordLen=8  CountFracLen=0  CountSampTime=1
      settings: SourceProductName=Simulink
  upper : simulink/Logic and Bit Operations/Compare To Constant  relop=<  const=(numTiles(1)-1)*dimTiles(1) + dimTiles(1)/2  OutDataTypeStr=boolean
  upperLowerCoutner : hdlsllib/Sources/HDL Counter  CountType=Count limited  CountInit=0  CountStep=1  CountMax=1  CountFromType=Initial value  CountFrom=0  CountResetPort=on  CountLoadPort=off  CountEnbPort=on  CountDirPort=off  CountDataType=Unsigned  CountWordLen=1  CountFracLen=0  CountSampTime=1
      settings: SourceProductName=Simulink
  leftIndex : Outport  VectorParamsAs1DForOutWhenUnconnected=off
  rightIndex : Outport  Port=2  VectorParamsAs1DForOutWhenUnconnected=off
  upperSignal : Outport  Port=3  VectorParamsAs1DForOutWhenUnconnected=off
  lowerSignal : Outport  Port=4  VectorParamsAs1DForOutWhenUnconnected=off
  colRevW : Outport  Port=5  VectorParamsAs1DForOutWhenUnconnected=off
  colW : Outport  Port=6  VectorParamsAs1DForOutWhenUnconnected=off
  rowRevW : Outport  Port=7  VectorParamsAs1DForOutWhenUnconnected=off
  rowW : Outport  Port=8  VectorParamsAs1DForOutWhenUnconnected=off
  normFactor : Outport  Port=9  VectorParamsAs1DForOutWhenUnconnected=off
  pipe1Done : Outport  Port=10  VectorParamsAs1DForOutWhenUnconnected=off
  pipe2Done : Outport  Port=11  VectorParamsAs1DForOutWhenUnconnected=off
  rdAddr : Outport  Port=12  VectorParamsAs1DForOutWhenUnconnected=off
  rdValid : Outport  Port=13  VectorParamsAs1DForOutWhenUnconnected=off
  busout : Outport  Port=14  VectorParamsAs1DForOutWhenUnconnected=off
  frameDone : Outport  Port=15  VectorParamsAs1DForOutWhenUnconnected=off
  wires:
  right/1 -> rightIndex/1
  Constant16/1 -> norm1/3
  Logical Operator3/1 -> Logical Operator16/2, leftRight/2
  Switch/1 -> colRevWCounter/2
  Add/1 -> right/3, left/1
  normFactorSw/1 -> normFactor/1
  Constant1/1 -> Product/2
  colWCounter/1 -> colRevWCounter/1, Data Type Conversion/1
  rowWCounter/1 -> rowRevWCounter/1, Data Type Conversion2/1
  Compare To Constant1/1 -> Logical Operator1/1, right/2
  Constant14/1 -> norm2/3
  bottom/1 -> Logical Operator/1, Logical Operator6/1, Logical Operator18/1, norm3/1, norm3/2
  colCounter/1 -> Compare To Constant2/1, For Each Subsystem/1(colCounter), Delay3/1
  Add1/1 -> rdAddr/1
  Constant15/1 -> norm1/1
  Constant3/1 -> For Each Subsystem/2(Index)
  rowRevWCounter/1 -> Data Type Conversion3/1
  Logical Operator1/1 -> Switch/2, norm1/2, norm2/2
  left/1 -> leftIndex/1
  leftRight/1 -> Compare To Constant1/1, Compare To Constant/1, Add/1, right/1, left/3
  For Each Subsystem/1(Out1) -> Logical Operator3/1
  Product/1 -> Delay1/1
  norm2/1 -> normFactorSw/3
  Constant13/1 -> norm2/1
  colRevWCounter/1 -> Data Type Conversion1/1
  Constant17/1 -> For Each Subsystem1/2(Index)
  Compare To Constant/1 -> Logical Operator1/2, left/2
  Constant5/1 -> Add/2
  Constant6/1 -> Switch/1
  Constant9/1 -> Switch1/3
  Logical Operator/1 -> normFactorSw/2, Switch1/2
  For Each Subsystem1/1(Out1) -> Logical Operator2/1
  Switch1/1 -> rowRevWCounter/2
  norm1/1 -> normFactorSw/1
  Constant8/1 -> Switch1/1
  Constant7/1 -> Switch/3
  pipe2/1 -> Compare To Constant4/1
  Compare To Constant4/1 -> Logical Operator5/1
  pipe1/1 -> Compare To Constant3/1
  Compare To Constant3/1 -> Logical Operator4/1
  Logical Operator4/1 -> Logical Operator6/2, Logical Operator7/1
  Logical Operator5/1 -> Logical Operator8/1, Logical Operator7/2
  Logical Operator6/1 -> Logical Operator9/1
  Logical Operator7/1 -> Logical Operator9/2
  Logical Operator8/1 -> Logical Operator9/3
  Logical Operator10/1 -> Logical Operator8/2
  Logical Operator9/1 -> colWCounter/2, colCounter/2, Delay2/1
  Logical Operator2/1 -> upperLowerCoutner/2, Logical Operator19/1
  Constant4/1 -> For Each Subsystem2/2(Index)
  For Each Subsystem2/1(Out1) -> Logical Operator11/1
  Logical Operator11/1 -> pipe1Done/1, Logical Operator15/1
  For Each Subsystem3/1(Out1) -> Logical Operator12/1
  Compare To Constant2/1 -> For Each Subsystem1/3(en), rowWCounter/2, For Each Subsystem2/3(en), Logical Operator13/1, For Each Subsystem3/3(en), Logical Operator16/1, leftRight/1, rowCounter/2
  Constant18/1 -> For Each Subsystem3/2(Index)
  rowCounter/1 -> Delay/1, upper/1, bottom/1, For Each Subsystem1/1(rowCounter), For Each Subsystem2/1(rowCounter), For Each Subsystem3/1(rowCounter), Compare To Constant5/1
  Switch2/1 -> Logical Operator15/2, pipe2Done/1
  Logical Operator12/1 -> Switch2/1
  Logical Operator13/1 -> Switch2/3
  Compare To Constant5/1 -> Logical Operator13/2
  HDL Counter1/1 -> Compare To Constant6/1
  HDL Counter/1 -> Compare To Constant8/1, Compare To Constant7/1
  Compare To Constant7/1 -> Logical Operator8/3, Logical Operator7/3
  Compare To Constant8/1 -> HDL Counter/1, HDL Counter1/1
  Compare To Constant6/1 -> Logical Operator14/1
  Logical Operator14/1 -> HDL Counter/2
  Logical Operator15/1 -> Logical Operator14/2, HDL Counter1/2
  Logical Operator16/1 -> colWCounter/1
  upper/1 -> Logical Operator10/1, Switch2/2, Logical Operator/2, Logical Operator18/2, norm3/3
  upperLowerCoutner/1 -> Compare To Constant9/1
  Compare To Constant9/1 -> norm4/1, Logical Operator17/1
  norm3/1 -> norm5/3, norm4/3
  norm5/1 -> lowerSignal/1
  norm4/1 -> upperSignal/1
  Logical Operator17/1 -> norm5/1
  Logical Operator18/1 -> norm5/2, norm4/2
  Data Type Conversion/1 -> colW/1
  Data Type Conversion1/1 -> colRevW/1
  Data Type Conversion2/1 -> rowW/1
  Data Type Conversion3/1 -> rowRevW/1
  Delay/1 -> Product/1
  Delay1/1 -> Add1/1
  Delay2/1 -> Delay11/1, rdValid/1
  Delay3/1 -> Add1/2
  Constant2/1 -> upperLowerCoutner/1, rowCounter/1, colCounter/1
  Delay11/1 -> pixelBusGenerator/1(validIn)
  pixelBusGenerator/1(busOut) -> busout/1
  pixelBusGenerator/2(frameDone) -> frameDone/1, Logical Operator19/2
  Logical Operator19/1 -> rowWCounter/1

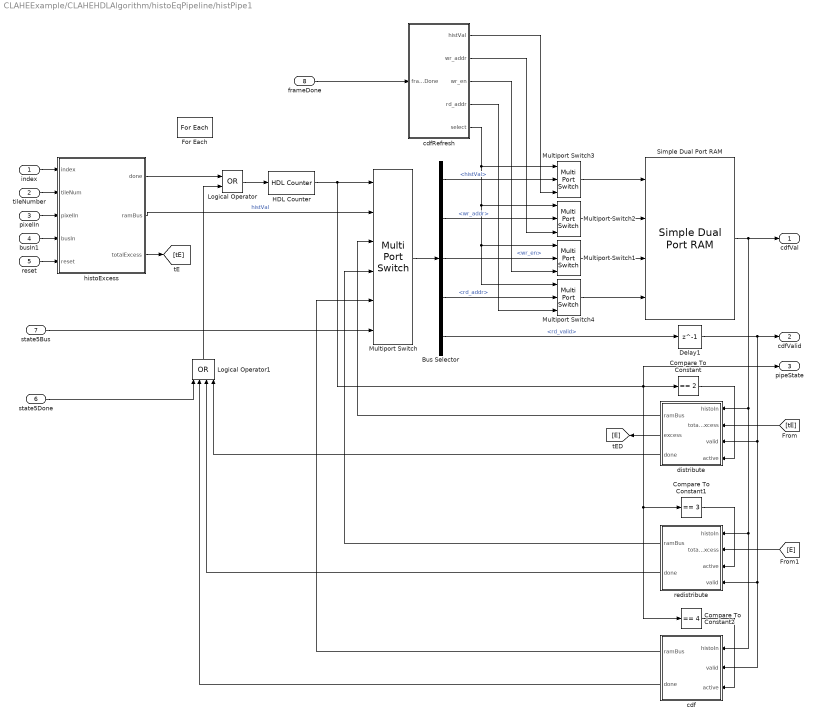
== system CLAHEExample/CLAHEHDLAlgorithm/histoEqPipeline/histPipe1 ==
  index : Inport  Partition=on  PartitionDimension=1  PartitionWidth=1  PartitionOffset=0
  tileNumber : Inport  Port=2
  pixelIn : Inport  Port=3
  busIn1 : Inport  Port=4
  reset : Inport  Port=5
  state5Done : Inport  Port=6
  state5Bus : Inport  Port=7
  frameDone : Inport  Port=8
  Bus Selector : BusSelector  OutputSignals=histVal,wr_addr,wr_en,rd_addr,rd_valid
  Compare To Constant : simulink/Logic and Bit Operations/Compare To Constant  relop===  const=2  OutDataTypeStr=boolean
  Compare To Constant1 : simulink/Logic and Bit Operations/Compare To Constant  relop===  const=3  OutDataTypeStr=boolean
  Compare To Constant2 : simulink/Logic and Bit Operations/Compare To Constant  relop===  const=4  OutDataTypeStr=boolean
  Delay1 : Delay  DelayLength=1
  For Each : ForEach  DisableCoverage=on
  HDL Counter : hdlsllib/Sources/HDL Counter  CountType=Count limited  CountInit=1  CountStep=1  CountMax=5  CountFromType=Initial value  CountFrom=1  CountResetPort=off  CountLoadPort=off  CountEnbPort=on  CountDirPort=off  CountDataType=Unsigned  CountWordLen=3  CountFracLen=0  CountSampTime=1
      settings: SourceProductName=Simulink
  Logical Operator : Logic  Operator=OR  AllPortsSameDT=off  OutDataTypeStr=boolean
  Logical Operator1 : Logic  Operator=OR  Inputs=4  AllPortsSameDT=off  OutDataTypeStr=boolean
  Multiport Switch : MultiPortSwitch  Inputs=5
  Multiport Switch{1..4} (4 alike) : MultiPortSwitch  Inputs=2
  Simple Dual Port RAM : hdlsllib/HDL RAMs/Simple Dual Port RAM  ram_size=ceil(log2(numBins-1))
      settings: SourceProductName=Simulink  SourceProductBaseCode=SL
  cdf : Subsystem
  cdfRefresh : Subsystem
  distribute : Subsystem
  histoExcess : Subsystem
  redistribute : Subsystem
  cdfVal : Outport  ConcatenationDimension=1  VectorParamsAs1DForOutWhenUnconnected=off
  cdfValid : Outport  Port=2  ConcatenationDimension=1  VectorParamsAs1DForOutWhenUnconnected=off
  pipeState : Outport  Port=3  ConcatenationDimension=1  VectorParamsAs1DForOutWhenUnconnected=off
  wires:
  pixelIn/1 -> histoExcess/3(pixelIn)
  busIn1/1 -> histoExcess/4(busIn)
  reset/1 -> histoExcess/5(reset)
  histoExcess/3(totalExcess) -> [tE]
  [tE] -> distribute/2(totalExcess)
  distribute/2(excess) -> [E]
  [E] -> redistribute/2(totalExcess)
  Multiport Switch/1 -> Bus Selector/1
  HDL Counter/1 -> Multiport Switch/1, Compare To Constant/1, pipeState/1, Compare To Constant2/1, Compare To Constant1/1
  histoExcess/2(ramBus) -> Multiport Switch/2  "histVal"
  Bus Selector/2 -> Multiport Switch2/2  "<wr_addr>"
  Bus Selector/3 -> Multiport Switch1/2  "<wr_en>"
  Bus Selector/4 -> Multiport Switch4/2  "<rd_addr>"
  Bus Selector/5 -> Delay1/1  "<rd_valid>"
  Delay1/1 -> cdfValid/1, cdf/2(valid), redistribute/4(valid), distribute/3(valid)
  Logical Operator/1 -> HDL Counter/1
  histoExcess/1(done) -> Logical Operator/1
  distribute/1(ramBus) -> Multiport Switch/3
  Compare To Constant/1 -> distribute/4(active)
  Compare To Constant1/1 -> redistribute/3(active)
  redistribute/1(ramBus) -> Multiport Switch/4
  Compare To Constant2/1 -> cdf/3(active)
  cdf/1(ramBus) -> Multiport Switch/5
  state5Bus/1 -> Multiport Switch/6
  Logical Operator1/1 -> Logical Operator/2
  state5Done/1 -> Logical Operator1/1
  redistribute/2(done) -> Logical Operator1/3
  cdf/2(done) -> Logical Operator1/2
  distribute/3(done) -> Logical Operator1/4
  Simple Dual Port RAM/1 -> cdfVal/1, cdf/1(histoIn), redistribute/1(histoIn), distribute/1(histoIn)
  index/1 -> histoExcess/1(index)
  tileNumber/1 -> histoExcess/2(tileNum)
  frameDone/1 -> cdfRefresh/1(frameDone)
  cdfRefresh/5(select) -> Multiport Switch2/1, Multiport Switch4/1, Multiport Switch1/1, Multiport Switch3/1
  cdfRefresh/3(wr_en) -> Multiport Switch1/3
  Bus Selector/1 -> Multiport Switch3/2  "<histVal>"
  cdfRefresh/1(histVal) -> Multiport Switch3/3
  cdfRefresh/2(wr_addr) -> Multiport Switch2/3
  cdfRefresh/4(rd_addr) -> Multiport Switch4/3
  Multiport Switch3/1 -> Simple Dual Port RAM/1
  Multiport Switch2/1 -> Simple Dual Port RAM/2
  Multiport Switch1/1 -> Simple Dual Port RAM/3
  Multiport Switch4/1 -> Simple Dual Port RAM/4

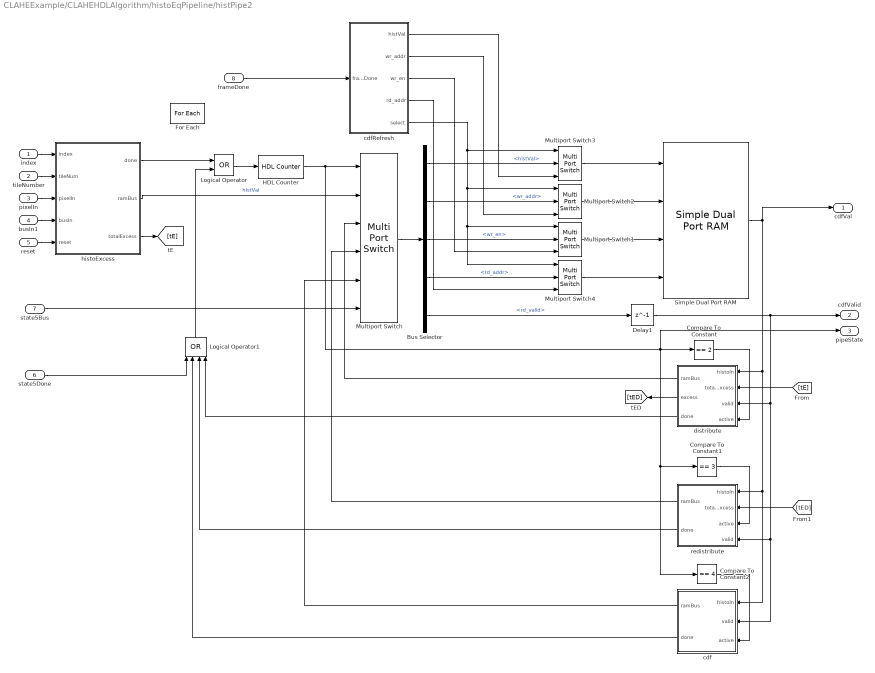
== system CLAHEExample/CLAHEHDLAlgorithm/histoEqPipeline/histPipe2 ==
  index : Inport  Partition=on  PartitionDimension=1  PartitionWidth=1  PartitionOffset=0
  tileNumber : Inport  Port=2
  pixelIn : Inport  Port=3
  busIn1 : Inport  Port=4
  reset : Inport  Port=5
  state5Done : Inport  Port=6
  state5Bus : Inport  Port=7
  frameDone : Inport  Port=8
  Bus Selector : BusSelector  OutputSignals=histVal,wr_addr,wr_en,rd_addr,rd_valid
  Compare To Constant : simulink/Logic and Bit Operations/Compare To Constant  relop===  const=2  OutDataTypeStr=boolean
  Compare To Constant1 : simulink/Logic and Bit Operations/Compare To Constant  relop===  const=3  OutDataTypeStr=boolean
  Compare To Constant2 : simulink/Logic and Bit Operations/Compare To Constant  relop===  const=4  OutDataTypeStr=boolean
  Delay1 : Delay  DelayLength=1
  For Each : ForEach  DisableCoverage=on
  HDL Counter : hdlsllib/Sources/HDL Counter  CountType=Count limited  CountInit=1  CountStep=1  CountMax=5  CountFromType=Initial value  CountFrom=1  CountResetPort=off  CountLoadPort=off  CountEnbPort=on  CountDirPort=off  CountDataType=Unsigned  CountWordLen=3  CountFracLen=0  CountSampTime=1
      settings: SourceProductName=Simulink
  Logical Operator : Logic  Operator=OR  AllPortsSameDT=off  OutDataTypeStr=boolean
  Logical Operator1 : Logic  Operator=OR  Inputs=4  AllPortsSameDT=off  OutDataTypeStr=boolean
  Multiport Switch : MultiPortSwitch  Inputs=5
  Multiport Switch{1..4} (4 alike) : MultiPortSwitch  Inputs=2
  Simple Dual Port RAM : hdlsllib/HDL RAMs/Simple Dual Port RAM  ram_size=ceil(log2(numBins-1))
      settings: SourceProductName=Simulink  SourceProductBaseCode=SL
  cdf : Subsystem
  cdfRefresh : Subsystem
  distribute : Subsystem
  histoExcess : Subsystem
  redistribute : Subsystem
  cdfVal : Outport  ConcatenationDimension=1  VectorParamsAs1DForOutWhenUnconnected=off
  cdfValid : Outport  Port=2  ConcatenationDimension=1  VectorParamsAs1DForOutWhenUnconnected=off
  pipeState : Outport  Port=3  ConcatenationDimension=1  VectorParamsAs1DForOutWhenUnconnected=off
  wires:
  pixelIn/1 -> histoExcess/3(pixelIn)
  busIn1/1 -> histoExcess/4(busIn)
  reset/1 -> histoExcess/5(reset)
  histoExcess/3(totalExcess) -> [tE]
  [tE] -> distribute/2(totalExcess)
  distribute/2(excess) -> [tED]
  [tED] -> redistribute/2(totalExcess)
  Multiport Switch/1 -> Bus Selector/1
  HDL Counter/1 -> Multiport Switch/1, pipeState/1, Compare To Constant/1, Compare To Constant2/1, Compare To Constant1/1
  histoExcess/2(ramBus) -> Multiport Switch/2  "histVal"
  Bus Selector/1 -> Multiport Switch3/2  "<histVal>"
  Bus Selector/2 -> Multiport Switch2/2  "<wr_addr>"
  Bus Selector/3 -> Multiport Switch1/2  "<wr_en>"
  Bus Selector/4 -> Multiport Switch4/2  "<rd_addr>"
  Bus Selector/5 -> Delay1/1  "<rd_valid>"
  Delay1/1 -> cdfValid/1, cdf/2(valid), redistribute/4(valid), distribute/3(valid)
  Logical Operator/1 -> HDL Counter/1
  histoExcess/1(done) -> Logical Operator/1
  distribute/1(ramBus) -> Multiport Switch/3
  Compare To Constant/1 -> distribute/4(active)
  Compare To Constant1/1 -> redistribute/3(active)
  redistribute/1(ramBus) -> Multiport Switch/4
  Compare To Constant2/1 -> cdf/3(active)
  cdf/1(ramBus) -> Multiport Switch/5
  state5Bus/1 -> Multiport Switch/6
  Logical Operator1/1 -> Logical Operator/2
  state5Done/1 -> Logical Operator1/1
  redistribute/2(done) -> Logical Operator1/3
  cdf/2(done) -> Logical Operator1/2
  distribute/3(done) -> Logical Operator1/4
  Simple Dual Port RAM/1 -> cdfVal/1, cdf/1(histoIn), redistribute/1(histoIn), distribute/1(histoIn)
  index/1 -> histoExcess/1(index)
  tileNumber/1 -> histoExcess/2(tileNum)
  frameDone/1 -> cdfRefresh/1(frameDone)
  cdfRefresh/5(select) -> Multiport Switch2/1, Multiport Switch4/1, Multiport Switch1/1, Multiport Switch3/1
  cdfRefresh/1(histVal) -> Multiport Switch3/3
  cdfRefresh/2(wr_addr) -> Multiport Switch2/3
  cdfRefresh/3(wr_en) -> Multiport Switch1/3
  cdfRefresh/4(rd_addr) -> Multiport Switch4/3
  Multiport Switch3/1 -> Simple Dual Port RAM/1
  Multiport Switch2/1 -> Simple Dual Port RAM/2
  Multiport Switch1/1 -> Simple Dual Port RAM/3
  Multiport Switch4/1 -> Simple Dual Port RAM/4
